simulink model "TST_PTLo_LosCalc"  (R2016b)
settings: Solver=FixedStepDiscrete  StartTime=0.0  StopTime=simTime  FixedStep=sampleTime  RelTol=1e-3
values from neighbouring files (symbols this model uses):
  testCase = 1    [initTST_PTLo_LosCalc_001.m]    (also in initTST_PTLo_LosCalc_002.m = 2)
libraries: simulink x3
settings Model: Creator=WF305  LastModifiedBy=WF305
settings DebuggingCC: SignalRangeChecking=error

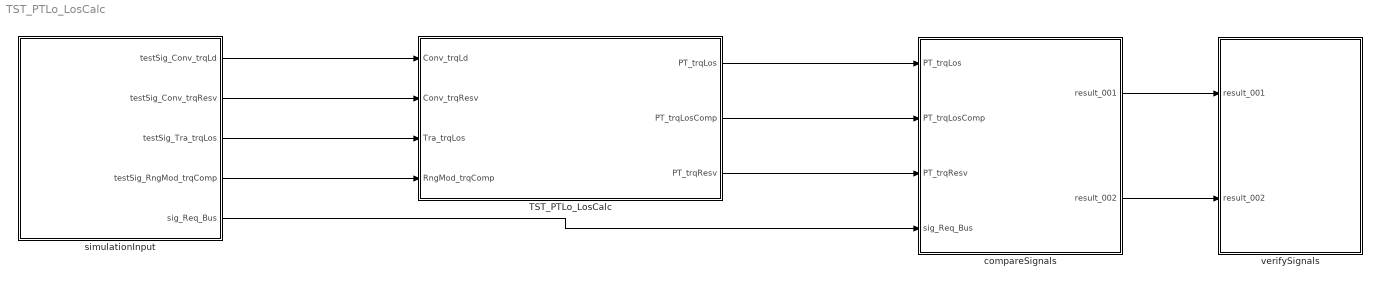
== system TST_PTLo_LosCalc ==
  TST_PTLo_LosCalc : Subsystem
  compareSignals : Subsystem
  simulationInput : Subsystem
  verifySignals : Subsystem
  wires:
  simulationInput/1(testSig_Conv_trqLd) -> TST_PTLo_LosCalc/1(Conv_trqLd)
  simulationInput/2(testSig_Conv_trqResv) -> TST_PTLo_LosCalc/2(Conv_trqResv)
  simulationInput/3(testSig_Tra_trqLos) -> TST_PTLo_LosCalc/3(Tra_trqLos)
  simulationInput/4(testSig_RngMod_trqComp) -> TST_PTLo_LosCalc/4(RngMod_trqComp)
  TST_PTLo_LosCalc/1(PT_trqLos) -> compareSignals/1(PT_trqLos)
  TST_PTLo_LosCalc/2(PT_trqLosComp) -> compareSignals/2(PT_trqLosComp)
  TST_PTLo_LosCalc/3(PT_trqResv) -> compareSignals/3(PT_trqResv)
  simulationInput/5(sig_Req_Bus) -> compareSignals/4(sig_Req_Bus)
  compareSignals/1(result_001) -> verifySignals/1(result_001)
  compareSignals/2(result_002) -> verifySignals/2(result_002)

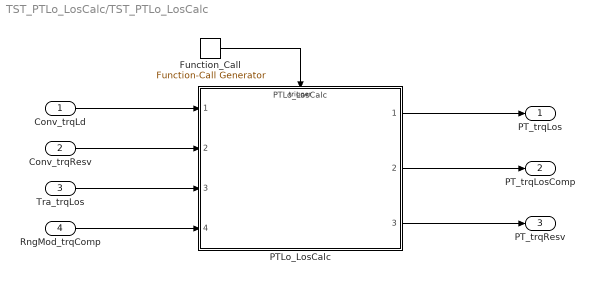
== system TST_PTLo_LosCalc/TST_PTLo_LosCalc ==
  Conv_trqLd : Inport
  Conv_trqResv : Inport  Port=2
  Tra_trqLos : Inport  Port=3
  RngMod_trqComp : Inport  Port=4
  Function_Call : simulink/Ports & Subsystems/Function-Call Generator  sample_time=sampleTime  numberOfIterations=1
  PTLo_LosCalc : ModelReference  ModelNameDialog=PTLo_LosCalc  ModelReferenceVersion=1.2  TriggerPortName=function  TriggerPortTriggerType=function-call  TriggerPortStatesWhenEnabling=held
  PT_trqLos : Outport
  PT_trqLosComp : Outport  Port=2
  PT_trqResv : Outport  Port=3
  wires:
  Function_Call/1 -> PTLo_LosCalc/Trigger
  Conv_trqLd/1 -> PTLo_LosCalc/1
  Conv_trqResv/1 -> PTLo_LosCalc/2
  Tra_trqLos/1 -> PTLo_LosCalc/3
  RngMod_trqComp/1 -> PTLo_LosCalc/4
  PTLo_LosCalc/1 -> PT_trqLos/1
  PTLo_LosCalc/2 -> PT_trqLosComp/1
  PTLo_LosCalc/3 -> PT_trqResv/1

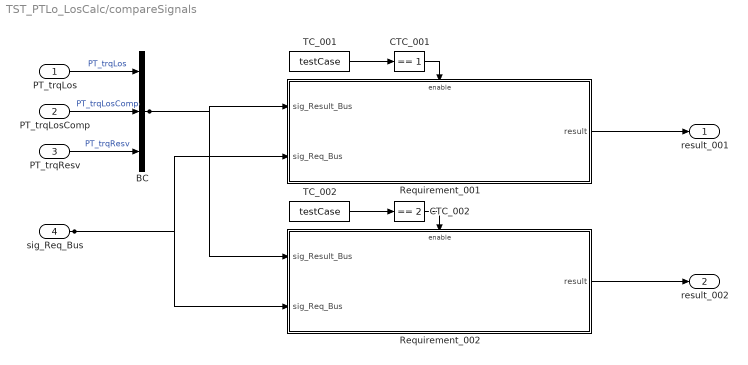
== system TST_PTLo_LosCalc/compareSignals ==
  PT_trqLos : Inport
  PT_trqLosComp : Inport  Port=2
  PT_trqResv : Inport  Port=3
  sig_Req_Bus : Inport  Port=4
  BC : BusCreator  Inputs=3
  CTC_001 : simulink/Logic and Bit Operations/Compare To Constant  relop===  const=1  OutDataTypeStr=boolean
  CTC_002 : simulink/Logic and Bit Operations/Compare To Constant  relop===  const=2  OutDataTypeStr=boolean
  Requirement_001 : Subsystem
  Requirement_002 : Subsystem
  TC_001 : Constant  Value=testCase
  TC_002 : Constant  Value=testCase
  result_001 : Outport
  result_002 : Outport  Port=2
  wires:
  PT_trqLos/1 -> BC/1  "PT_trqLos"
  PT_trqLosComp/1 -> BC/2  "PT_trqLosComp"
  PT_trqResv/1 -> BC/3  "PT_trqResv"
  TC_001/1 -> CTC_001/1
  CTC_001/1 -> Requirement_001/Enable
  sig_Req_Bus/1 -> Requirement_001/2(sig_Req_Bus), Requirement_002/2(sig_Req_Bus)
  BC/1 -> Requirement_001/1(sig_Result_Bus), Requirement_002/1(sig_Result_Bus)
  Requirement_001/1(result) -> result_001/1
  TC_002/1 -> CTC_002/1
  CTC_002/1 -> Requirement_002/Enable
  Requirement_002/1(result) -> result_002/1

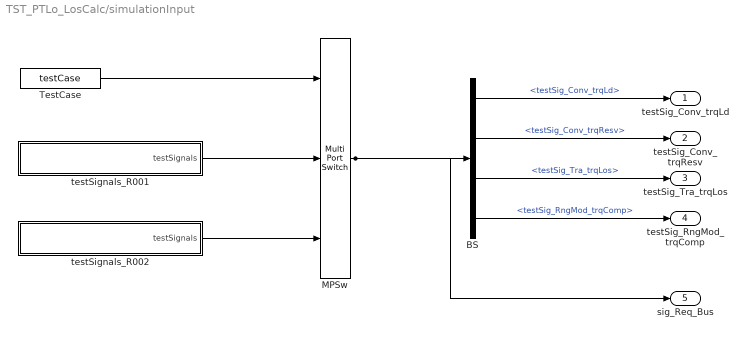
== system TST_PTLo_LosCalc/simulationInput ==
  BS : BusSelector  OutputSignals=testSig_Conv_trqLd,testSig_Conv_trqResv,testSig_Tra_trqLos,testSig_RngMod_trqComp
  MPSw : MultiPortSwitch  Inputs=2  SaturateOnIntegerOverflow=on  InputSameDT=on
  TestCase : Constant  Value=testCase
  testSignals_R001 : Subsystem
  testSignals_R002 : Subsystem
  testSig_Conv_trqLd : Outport
  testSig_Conv_trqResv : Outport  Port=2
  testSig_Tra_trqLos : Outport  Port=3
  testSig_RngMod_trqComp : Outport  Port=4
  sig_Req_Bus : Outport  Port=5
  wires:
  BS/1 -> testSig_Conv_trqLd/1  "<testSig_Conv_trqLd>"
  BS/2 -> testSig_Conv_trqResv/1  "<testSig_Conv_trqResv>"
  BS/3 -> testSig_Tra_trqLos/1  "<testSig_Tra_trqLos>"
  BS/4 -> testSig_RngMod_trqComp/1  "<testSig_RngMod_trqComp>"
  MPSw/1 -> BS/1, sig_Req_Bus/1
  TestCase/1 -> MPSw/1
  testSignals_R001/1(testSignals) -> MPSw/2
  testSignals_R002/1(testSignals) -> MPSw/3

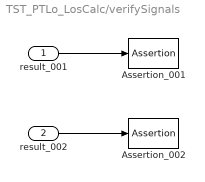
== system TST_PTLo_LosCalc/verifySignals ==
  result_001 : Inport
  result_002 : Inport  Port=2
  Assertion_001 : Assertion  Enabled=off
  Assertion_002 : Assertion  Enabled=off
  wires:
  result_001/1 -> Assertion_001/1
  result_002/1 -> Assertion_002/1

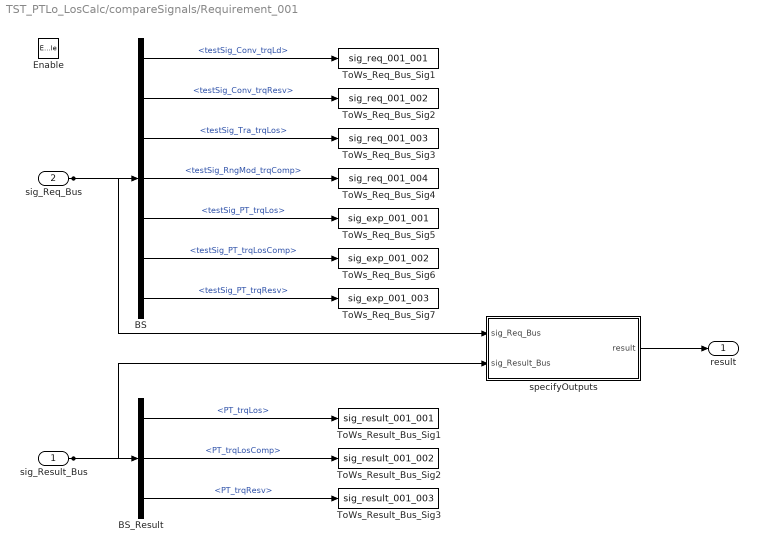
== system TST_PTLo_LosCalc/compareSignals/Requirement_001 ==
  sig_Result_Bus : Inport
  sig_Req_Bus : Inport  Port=2
  Enable : EnablePort
  BS : BusSelector  OutputSignals=testSig_Conv_trqLd,testSig_Conv_trqResv,testSig_Tra_trqLos,testSig_RngMod_trqComp,testSig_PT_trqLos,testSig_PT_trqLosComp,testSig_PT_trqResv
  BS_Result : BusSelector  OutputSignals=PT_trqLos,PT_trqLosComp,PT_trqResv
  ToWs_Req_Bus_Sig1 : ToWorkspace  VariableName=sig_req_001_001  SaveFormat=Structure With Time
  ToWs_Req_Bus_Sig2 : ToWorkspace  VariableName=sig_req_001_002  SaveFormat=Structure With Time
  ToWs_Req_Bus_Sig3 : ToWorkspace  VariableName=sig_req_001_003  SaveFormat=Structure With Time
  ToWs_Req_Bus_Sig4 : ToWorkspace  VariableName=sig_req_001_004  SaveFormat=Structure With Time
  ToWs_Req_Bus_Sig5 : ToWorkspace  VariableName=sig_exp_001_001  SaveFormat=Structure With Time
  ToWs_Req_Bus_Sig6 : ToWorkspace  VariableName=sig_exp_001_002  SaveFormat=Structure With Time
  ToWs_Req_Bus_Sig7 : ToWorkspace  VariableName=sig_exp_001_003  SaveFormat=Structure With Time
  ToWs_Result_Bus_Sig1 : ToWorkspace  VariableName=sig_result_001_001  SaveFormat=Structure With Time
  ToWs_Result_Bus_Sig2 : ToWorkspace  VariableName=sig_result_001_002  SaveFormat=Structure With Time
  ToWs_Result_Bus_Sig3 : ToWorkspace  VariableName=sig_result_001_003  SaveFormat=Structure With Time
  specifyOutputs : Subsystem
  result : Outport
  wires:
  sig_Req_Bus/1 -> BS/1, specifyOutputs/1(sig_Req_Bus)
  BS/1 -> ToWs_Req_Bus_Sig1/1  "<testSig_Conv_trqLd>"
  BS/2 -> ToWs_Req_Bus_Sig2/1  "<testSig_Conv_trqResv>"
  BS/3 -> ToWs_Req_Bus_Sig3/1  "<testSig_Tra_trqLos>"
  BS/4 -> ToWs_Req_Bus_Sig4/1  "<testSig_RngMod_trqComp>"
  BS/5 -> ToWs_Req_Bus_Sig5/1  "<testSig_PT_trqLos>"
  BS/6 -> ToWs_Req_Bus_Sig6/1  "<testSig_PT_trqLosComp>"
  BS/7 -> ToWs_Req_Bus_Sig7/1  "<testSig_PT_trqResv>"
  sig_Result_Bus/1 -> BS_Result/1, specifyOutputs/2(sig_Result_Bus)
  BS_Result/1 -> ToWs_Result_Bus_Sig1/1  "<PT_trqLos>"
  BS_Result/2 -> ToWs_Result_Bus_Sig2/1  "<PT_trqLosComp>"
  BS_Result/3 -> ToWs_Result_Bus_Sig3/1  "<PT_trqResv>"
  specifyOutputs/1(result) -> result/1

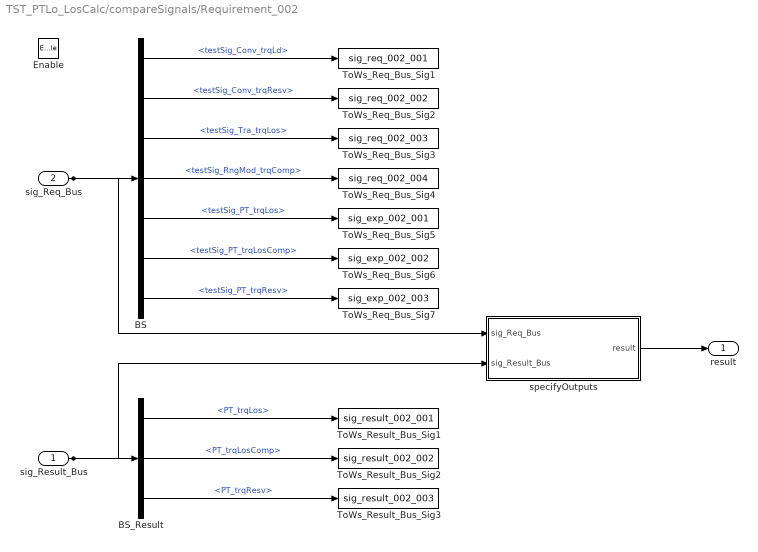
== system TST_PTLo_LosCalc/compareSignals/Requirement_002 ==
  sig_Result_Bus : Inport
  sig_Req_Bus : Inport  Port=2
  Enable : EnablePort
  BS : BusSelector  OutputSignals=testSig_Conv_trqLd,testSig_Conv_trqResv,testSig_Tra_trqLos,testSig_RngMod_trqComp,testSig_PT_trqLos,testSig_PT_trqLosComp,testSig_PT_trqResv
  BS_Result : BusSelector  OutputSignals=PT_trqLos,PT_trqLosComp,PT_trqResv
  ToWs_Req_Bus_Sig1 : ToWorkspace  VariableName=sig_req_002_001  SaveFormat=Structure With Time
  ToWs_Req_Bus_Sig2 : ToWorkspace  VariableName=sig_req_002_002  SaveFormat=Structure With Time
  ToWs_Req_Bus_Sig3 : ToWorkspace  VariableName=sig_req_002_003  SaveFormat=Structure With Time
  ToWs_Req_Bus_Sig4 : ToWorkspace  VariableName=sig_req_002_004  SaveFormat=Structure With Time
  ToWs_Req_Bus_Sig5 : ToWorkspace  VariableName=sig_exp_002_001  SaveFormat=Structure With Time
  ToWs_Req_Bus_Sig6 : ToWorkspace  VariableName=sig_exp_002_002  SaveFormat=Structure With Time
  ToWs_Req_Bus_Sig7 : ToWorkspace  VariableName=sig_exp_002_003  SaveFormat=Structure With Time
  ToWs_Result_Bus_Sig1 : ToWorkspace  VariableName=sig_result_002_001  SaveFormat=Structure With Time
  ToWs_Result_Bus_Sig2 : ToWorkspace  VariableName=sig_result_002_002  SaveFormat=Structure With Time
  ToWs_Result_Bus_Sig3 : ToWorkspace  VariableName=sig_result_002_003  SaveFormat=Structure With Time
  specifyOutputs : Subsystem
  result : Outport
  wires:
  sig_Req_Bus/1 -> BS/1, specifyOutputs/1(sig_Req_Bus)
  BS/1 -> ToWs_Req_Bus_Sig1/1  "<testSig_Conv_trqLd>"
  BS/2 -> ToWs_Req_Bus_Sig2/1  "<testSig_Conv_trqResv>"
  BS/3 -> ToWs_Req_Bus_Sig3/1  "<testSig_Tra_trqLos>"
  BS/4 -> ToWs_Req_Bus_Sig4/1  "<testSig_RngMod_trqComp>"
  BS/5 -> ToWs_Req_Bus_Sig5/1  "<testSig_PT_trqLos>"
  BS/6 -> ToWs_Req_Bus_Sig6/1  "<testSig_PT_trqLosComp>"
  BS/7 -> ToWs_Req_Bus_Sig7/1  "<testSig_PT_trqResv>"
  sig_Result_Bus/1 -> BS_Result/1, specifyOutputs/2(sig_Result_Bus)
  BS_Result/1 -> ToWs_Result_Bus_Sig1/1  "<PT_trqLos>"
  BS_Result/2 -> ToWs_Result_Bus_Sig2/1  "<PT_trqLosComp>"
  BS_Result/3 -> ToWs_Result_Bus_Sig3/1  "<PT_trqResv>"
  specifyOutputs/1(result) -> result/1

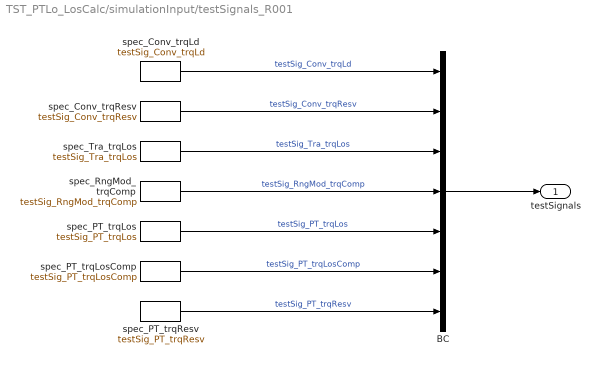
== system TST_PTLo_LosCalc/simulationInput/testSignals_R001 ==
  BC : BusCreator  Inputs=7
  spec_Conv_trqLd : FromWorkspace  VariableName=testSig_Conv_trqLd  Interpolate=off  OutputAfterFinalValue=Holding final value
  spec_Conv_trqResv : FromWorkspace  VariableName=testSig_Conv_trqResv  Interpolate=off  OutputAfterFinalValue=Holding final value
  spec_PT_trqLos : FromWorkspace  VariableName=testSig_PT_trqLos  Interpolate=off  OutputAfterFinalValue=Holding final value
  spec_PT_trqLosComp : FromWorkspace  VariableName=testSig_PT_trqLosComp  Interpolate=off  OutputAfterFinalValue=Holding final value
  spec_PT_trqResv : FromWorkspace  VariableName=testSig_PT_trqResv  Interpolate=off  OutputAfterFinalValue=Holding final value
  spec_RngMod_trqComp : FromWorkspace  VariableName=testSig_RngMod_trqComp  Interpolate=off  OutputAfterFinalValue=Holding final value
  spec_Tra_trqLos : FromWorkspace  VariableName=testSig_Tra_trqLos  Interpolate=off  OutputAfterFinalValue=Holding final value
  testSignals : Outport
  wires:
  BC/1 -> testSignals/1
  spec_Conv_trqLd/1 -> BC/1  "testSig_Conv_trqLd"
  spec_Conv_trqResv/1 -> BC/2  "testSig_Conv_trqResv"
  spec_Tra_trqLos/1 -> BC/3  "testSig_Tra_trqLos"
  spec_RngMod_trqComp/1 -> BC/4  "testSig_RngMod_trqComp"
  spec_PT_trqLos/1 -> BC/5  "testSig_PT_trqLos"
  spec_PT_trqLosComp/1 -> BC/6  "testSig_PT_trqLosComp"
  spec_PT_trqResv/1 -> BC/7  "testSig_PT_trqResv"

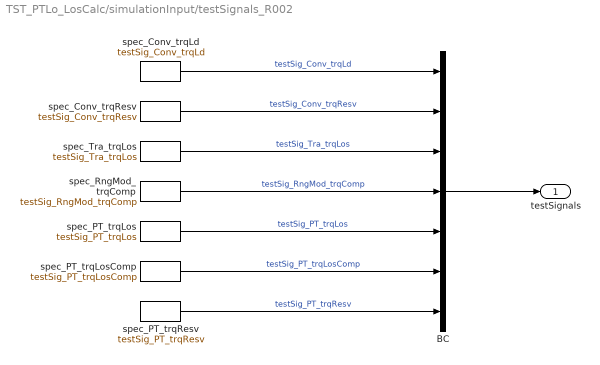
== system TST_PTLo_LosCalc/simulationInput/testSignals_R002 ==
  BC : BusCreator  Inputs=7
  spec_Conv_trqLd : FromWorkspace  VariableName=testSig_Conv_trqLd  Interpolate=off  OutputAfterFinalValue=Holding final value
  spec_Conv_trqResv : FromWorkspace  VariableName=testSig_Conv_trqResv  Interpolate=off  OutputAfterFinalValue=Holding final value
  spec_PT_trqLos : FromWorkspace  VariableName=testSig_PT_trqLos  Interpolate=off  OutputAfterFinalValue=Holding final value
  spec_PT_trqLosComp : FromWorkspace  VariableName=testSig_PT_trqLosComp  Interpolate=off  OutputAfterFinalValue=Holding final value
  spec_PT_trqResv : FromWorkspace  VariableName=testSig_PT_trqResv  Interpolate=off  OutputAfterFinalValue=Holding final value
  spec_RngMod_trqComp : FromWorkspace  VariableName=testSig_RngMod_trqComp  Interpolate=off  OutputAfterFinalValue=Holding final value
  spec_Tra_trqLos : FromWorkspace  VariableName=testSig_Tra_trqLos  Interpolate=off  OutputAfterFinalValue=Holding final value
  testSignals : Outport
  wires:
  BC/1 -> testSignals/1
  spec_Conv_trqLd/1 -> BC/1  "testSig_Conv_trqLd"
  spec_Conv_trqResv/1 -> BC/2  "testSig_Conv_trqResv"
  spec_Tra_trqLos/1 -> BC/3  "testSig_Tra_trqLos"
  spec_RngMod_trqComp/1 -> BC/4  "testSig_RngMod_trqComp"
  spec_PT_trqLos/1 -> BC/5  "testSig_PT_trqLos"
  spec_PT_trqLosComp/1 -> BC/6  "testSig_PT_trqLosComp"
  spec_PT_trqResv/1 -> BC/7  "testSig_PT_trqResv"

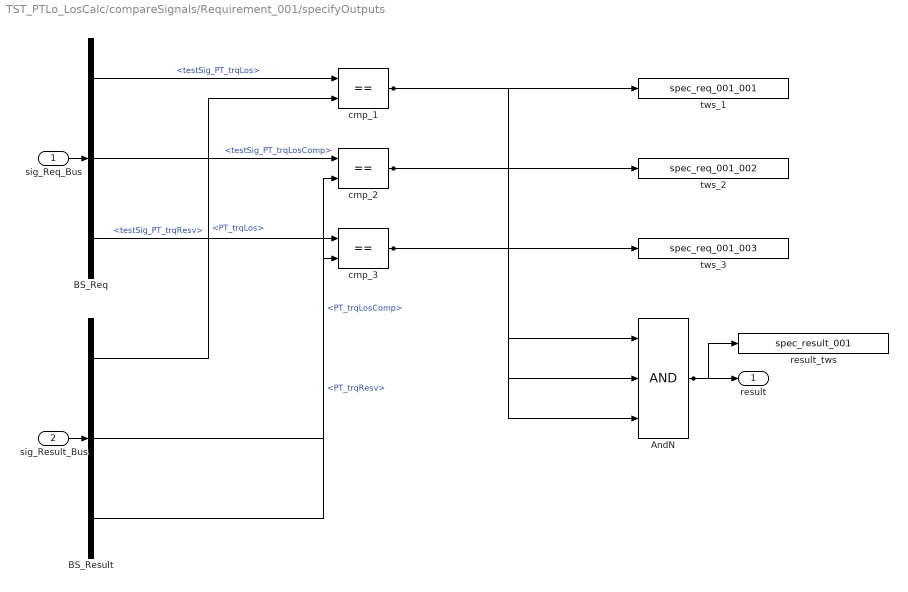
== system TST_PTLo_LosCalc/compareSignals/Requirement_001/specifyOutputs ==
  sig_Req_Bus : Inport
  sig_Result_Bus : Inport  Port=2
  AndN : Logic  Inputs=3
  BS_Req : BusSelector  OutputSignals=testSig_PT_trqLos,testSig_PT_trqLosComp,testSig_PT_trqResv
  BS_Result : BusSelector  OutputSignals=PT_trqLos,PT_trqLosComp,PT_trqResv
  cmp_1 : RelationalOperator  Operator===  RndMeth=Nearest  InputSameDT=on
  cmp_2 : RelationalOperator  Operator===  RndMeth=Nearest  InputSameDT=on
  cmp_3 : RelationalOperator  Operator===  RndMeth=Nearest  InputSameDT=on
  result_tws : ToWorkspace  VariableName=spec_result_001
  tws_1 : ToWorkspace  VariableName=spec_req_001_001
  tws_2 : ToWorkspace  VariableName=spec_req_001_002
  tws_3 : ToWorkspace  VariableName=spec_req_001_003
  result : Outport
  wires:
  sig_Req_Bus/1 -> BS_Req/1
  sig_Result_Bus/1 -> BS_Result/1
  AndN/1 -> result/1, result_tws/1
  BS_Req/1 -> cmp_1/1  "<testSig_PT_trqLos>"
  BS_Result/1 -> cmp_1/2  "<PT_trqLos>"
  cmp_1/1 -> tws_1/1, AndN/1
  BS_Req/2 -> cmp_2/1  "<testSig_PT_trqLosComp>"
  BS_Result/2 -> cmp_2/2  "<PT_trqLosComp>"
  cmp_2/1 -> tws_2/1, AndN/2
  BS_Req/3 -> cmp_3/1  "<testSig_PT_trqResv>"
  BS_Result/3 -> cmp_3/2  "<PT_trqResv>"
  cmp_3/1 -> tws_3/1, AndN/3

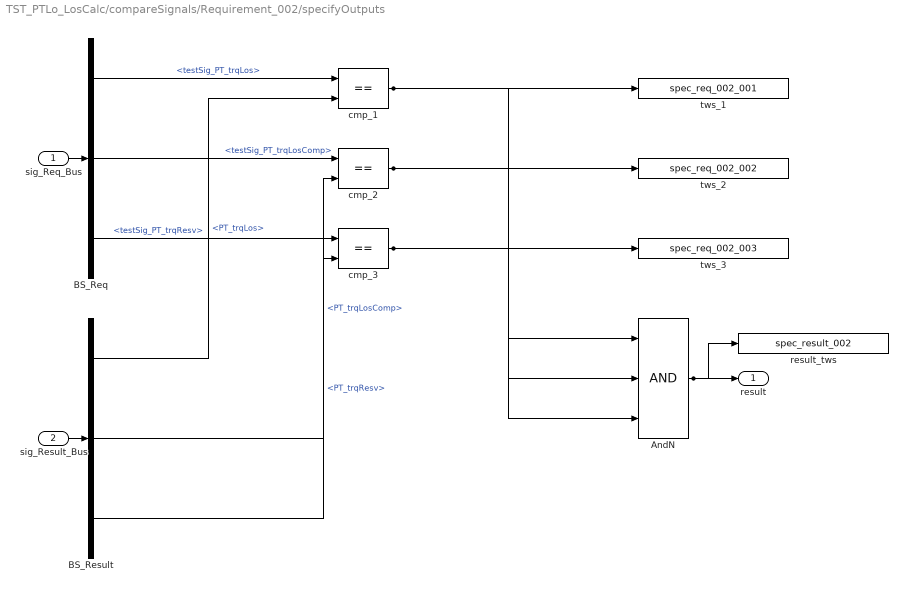
== system TST_PTLo_LosCalc/compareSignals/Requirement_002/specifyOutputs ==
  sig_Req_Bus : Inport
  sig_Result_Bus : Inport  Port=2
  AndN : Logic  Inputs=3
  BS_Req : BusSelector  OutputSignals=testSig_PT_trqLos,testSig_PT_trqLosComp,testSig_PT_trqResv
  BS_Result : BusSelector  OutputSignals=PT_trqLos,PT_trqLosComp,PT_trqResv
  cmp_1 : RelationalOperator  Operator===  RndMeth=Nearest  InputSameDT=on
  cmp_2 : RelationalOperator  Operator===  RndMeth=Nearest  InputSameDT=on
  cmp_3 : RelationalOperator  Operator===  RndMeth=Nearest  InputSameDT=on
  result_tws : ToWorkspace  VariableName=spec_result_002
  tws_1 : ToWorkspace  VariableName=spec_req_002_001
  tws_2 : ToWorkspace  VariableName=spec_req_002_002
  tws_3 : ToWorkspace  VariableName=spec_req_002_003
  result : Outport
  wires:
  sig_Req_Bus/1 -> BS_Req/1
  sig_Result_Bus/1 -> BS_Result/1
  AndN/1 -> result/1, result_tws/1
  BS_Req/1 -> cmp_1/1  "<testSig_PT_trqLos>"
  BS_Result/1 -> cmp_1/2  "<PT_trqLos>"
  cmp_1/1 -> tws_1/1, AndN/1
  BS_Req/2 -> cmp_2/1  "<testSig_PT_trqLosComp>"
  BS_Result/2 -> cmp_2/2  "<PT_trqLosComp>"
  cmp_2/1 -> tws_2/1, AndN/2
  BS_Req/3 -> cmp_3/1  "<testSig_PT_trqResv>"
  BS_Result/3 -> cmp_3/2  "<PT_trqResv>"
  cmp_3/1 -> tws_3/1, AndN/3
